simulink model "cruise_control"  (R2026a)
settings: Solver=VariableStepAuto  StopTime=100.0
values from neighbouring files (symbols this model uses):
  A = 2.2    [init.m]
  Cd = 0.3    [init.m]
  Kd = Kd_range(k)    [controller_optimizer.m]    (also in init.m = 0)
  Ki = Ki_range(j)    [controller_optimizer.m]    (also in init.m = 10)
  Kp = Kp_range(i)    [controller_optimizer.m]    (also in init.m = 100)
  m = 1500.0    (= 1500)    [init.m]
  rho = 1.225    [init.m]
  v_ref = 30.0    (= 30)    [analyze_results.m]    (also in init.m)
libraries: slpidlib x1
settings Model: Creator=korki  LastModifiedBy=korki

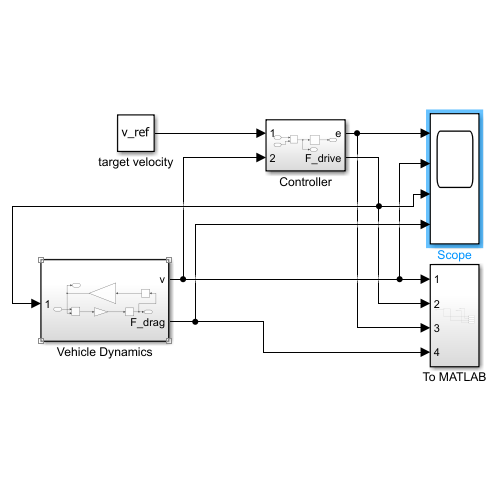
[thumbnail: Simulink's stored preview of the top-level diagram]
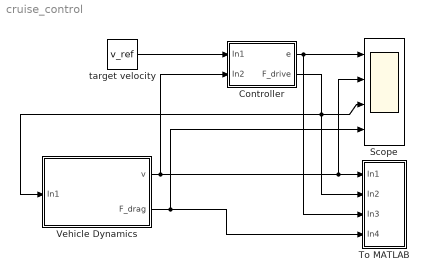
== system cruise_control ==
  Controller : Subsystem
  Scope : Scope  NumInputPorts=4
      settings: ActiveDisplayYMinimum=-12.966734807536643  ActiveDisplayYMaximum=34.774081645281846
  To MATLAB : Subsystem
  Vehicle Dynamics : Subsystem
  target velocity : Constant  Value=v_ref
  wires:
  Controller/2(F_drive) -> Scope/3, Vehicle Dynamics/1(In1), To MATLAB/2(In2)
  target velocity/1 -> Controller/1(In1)
  Vehicle Dynamics/1(v) -> Scope/2, To MATLAB/1(In1), Controller/2(In2)
  Vehicle Dynamics/2(F_drag) -> Scope/4, To MATLAB/4(In4)
  Controller/1(e) -> Scope/1, To MATLAB/3(In3)

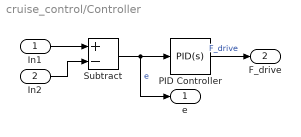
== system cruise_control/Controller ==
  In1 : Inport
  In2 : Inport  Port=2
  PID Controller : slpidlib/PID Controller  Controller=PID  Form=Parallel  TimeDomain=Continuous-time  UseExternalTs=off  SampleTime=-1  IntegratorMethod=Forward Euler  FilterMethod=Forward Euler  ControllerParametersSource=internal  P=Kp  I=Ki  UseKiTs=off  D=Kd  UseExternalDerivativeSource=off  N=100  UseFilter=on  TunerSelectOption=Transfer Function Based (PID Tuner App)  InitialConditionSource=internal  InitialConditionForIntegrator=0  InitialConditionForFilter=0  DifferentiatorICPrevScaledInput=0  ExternalReset=none  TrackingMode=off  Kt=1  LimitOutput=off  SatLimitsSource=internal  UpperSaturationLimit=inf  LowerSaturationLimit=-inf  LinearizeAsGain=on  AntiWindupMode=none  Kb=1  LimitIntegrator=off  UpperIntegratorSaturationLimit=inf  LowerIntegratorSaturationLimit=-inf  POutMin=[]  POutMax=[]  IOutMin=[]  IOutMax=[]  DOutMin=[]  DOutMax=[]  NOutMin=[]  NOutMax=[]  SumOutMin=[]  SumOutMax=[]  SaturationOutMin=[]  SaturationOutMax=[]  PParamMin=[]  PParamMax=[]  IParamMin=[]  IParamMax=[]  DParamMin=[]  DParamMax=[]  NParamMin=[]  NParamMax=[]  KbParamMin=[]  KbParamMax=[]  KtParamMin=[]  KtParamMax=[]  KbOutMin=[]  KbOutMax=[]  KtOutMin=[]  KtOutMax=[]  IntegratorOutMin=[]  IntegratorOutMax=[]  FilterOutMin=[]  FilterOutMax=[]  SumI1OutMin=[]  SumI1OutMax=[]  SumI2OutMin=[]  SumI2OutMax=[]  SumI3OutMin=[]  SumI3OutMax=[]  SumI4OutMin=[]  SumI4OutMax=[]  SumDOutMin=[]  SumDOutMax=[]  DifferentiatorOutMin=[]  DifferentiatorOutMax=[]  FilterDiffOutCoefMin=[]  FilterDiffOutCoefMax=[]  ReciprocalOutMin=[]  ReciprocalOutMax=[]  SumDenOutMin=[]  SumDenOutMax=[]  SumNumOutMin=[]  SumNumOutMax=[]  DivideOutMin=[]  DivideOutMax=[]  UdiffTsProdOutMin=[]  UdiffTsProdOutMax=[]  NTsProdOutMin=[]  NTsProdOutMax=[]  UintegralTsProdOutMin=[]  UintegralTsProdOutMax=[]  UngainTsProdOutMin=[]  UngainTsProdOutMax=[]  ClampingZeroOutDataTypeStr=Inherit: Inherit via back propagation  ClampingZeroOutMin=[]  ClampingZeroOutMax=[]  FilterDenConstantOutDataTypeStr=Inherit: Inherit via back propagation  FilterDenConstantOutMin=[]  FilterDenConstantOutMax=[]  PCopyOutDataTypeStr=Inherit: Inherit via back propagation  PCopyOutMin=[]  PCopyOutMax=[]  NCopyOutDataTypeStr=Inherit: Inherit via back propagation  NCopyOutMin=[]  NCopyOutMax=[]  IntegratorContinuousStateAttributes=''  IntegratorStateMustResolveToSignalObject=off  IntegratorRTWStateStorageClass=Auto  FilterContinuousStateAttributes=''  FilterStateMustResolveToSignalObject=off  FilterRTWStateStorageClass=Auto  ParallelPVariant=InternalParameters  IdealPVariant=Disabled  IVariant=InternalParameters  DVariant=InternalParameters  IntegratorVariant=Continuous  SatVariant=Disabled  AWVariant=Passthrough  PCopyVariant=Disabled  TRVariant=Disabled  FdbkBlocksVariant=Forward  IdealPFdbkVariant=Disabled  SatFdbkVariant=Disabled  DerivativeFilterVariant=ContFilter  NVariant=InternalParameters  NCopyVariant=Disabled  FilterICVariant=InternalICsFilter  IntegratorICVariant=InternalICs  ExternalResetVariant=Disabled  TRSumVariant=Passthrough  SumFdbkVariant=Disabled  SumVariant=Sum_PID  TsampFilterVariant=InternalTs  TsampNgainVariant=Passthrough  TsampIntegralVariant=Disabled_SignalSpec  ExternalSaturationOutDataTypeStr=Inherit: Same as second input  DerivativeSourceVariant=ErrorSignal  PreIntVariant=InternalPreInt
  Subtract : Sum  Inputs=+-
  e : Outport
  F_drive : Outport  Port=2
  wires:
  PID Controller/1 -> F_drive/1  "F_drive"
  In1/1 -> Subtract/1
  In2/1 -> Subtract/2
  Subtract/1 -> e/1, PID Controller/1  "e"

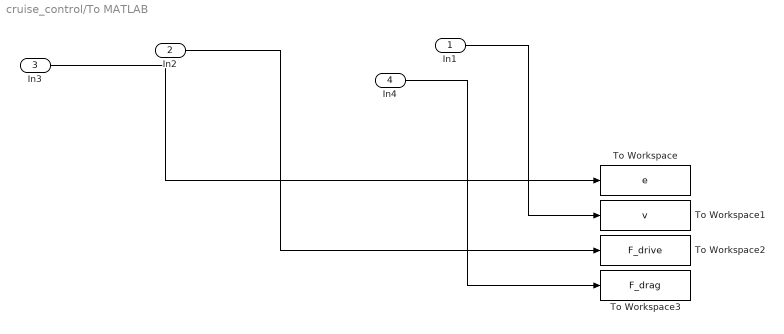
== system cruise_control/To MATLAB ==
  In1 : Inport
  In2 : Inport  Port=2
  In3 : Inport  Port=3
  In4 : Inport  Port=4
  To Workspace : ToWorkspace  VariableName=e  SaveFormat=Timeseries  SampleTime=-1
  To Workspace1 : ToWorkspace  VariableName=v  SaveFormat=Timeseries  SampleTime=-1
  To Workspace2 : ToWorkspace  VariableName=F_drive  SaveFormat=Timeseries  SampleTime=-1
  To Workspace3 : ToWorkspace  VariableName=F_drag  SaveFormat=Timeseries  SampleTime=-1
  wires:
  In3/1 -> To Workspace/1
  In1/1 -> To Workspace1/1
  In4/1 -> To Workspace3/1
  In2/1 -> To Workspace2/1

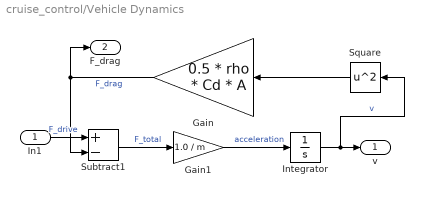
== system cruise_control/Vehicle Dynamics ==
  In1 : Inport
  Gain : Gain  Gain=0.5 * rho * Cd * A
  Gain1 : Gain  Gain=1.0 / m
  Integrator : Integrator
  Square : Math  Operator=square
  Subtract1 : Sum  Inputs=+-
  v : Outport
  F_drag : Outport  Port=2
  wires:
  In1/1 -> Subtract1/1  "F_drive"
  Square/1 -> Gain/1
  Integrator/1 -> Square/1, v/1  "v"
  Subtract1/1 -> Gain1/1  "F_total"
  Gain/1 -> Subtract1/2, F_drag/1  "F_drag"
  Gain1/1 -> Integrator/1  "acceleration"
